simulink model "Model02"  (R2018a)
settings: Solver=VariableStepAuto  StartTime=0.0  StopTime=10.0  RelTol=1e-3
undefined symbols (not defined in the file or in its folder): b, k, m
settings Model: Creator=ameli  LastModifiedBy=ameli
settings DataIOCC: Refine=10

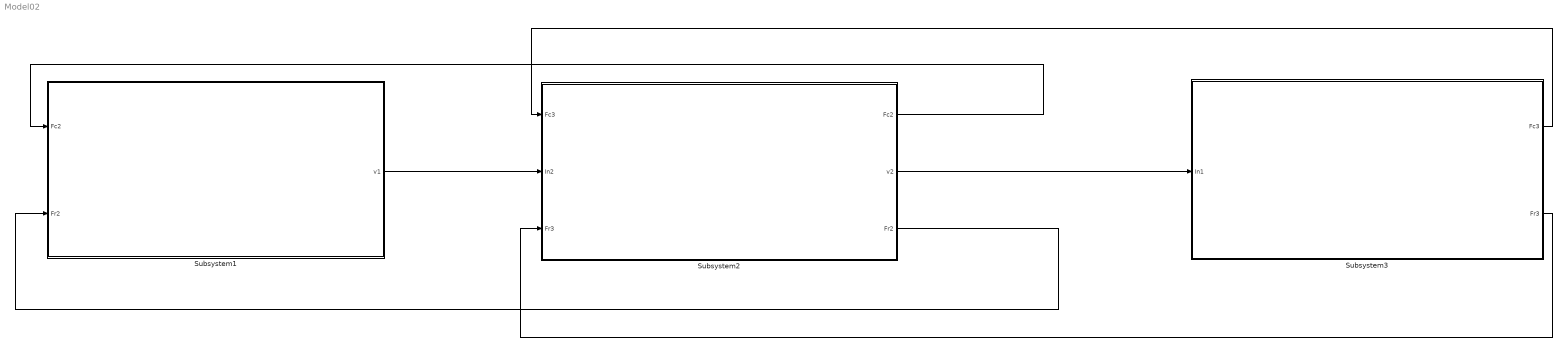
== system Model02 ==
  "Subsystem1 " : Subsystem
  Subsystem2 : Subsystem
  Subsystem3 : Subsystem
  wires:
  Subsystem3/2(Fr3) -> Subsystem2/3(Fr3)
  Subsystem2/3(Fr2) -> "Subsystem1 "/2(Fr2)
  Subsystem3/1(Fc3) -> Subsystem2/1(Fc3)
  Subsystem2/1(Fc2) -> "Subsystem1 "/1(Fc2)
  "Subsystem1 "/1(v1) -> Subsystem2/2(In2)
  Subsystem2/2(v2) -> Subsystem3/1(In1)

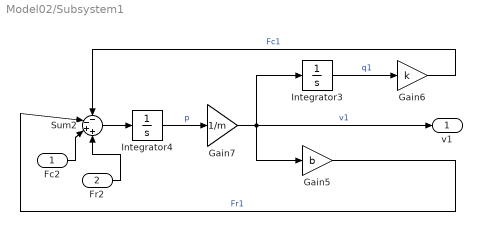
== system Model02/Subsystem1  ==
  Fc2 : Inport
  Fr2 : Inport  Port=2
  Gain5 : Gain  Gain=b
  Gain6 : Gain  Gain=k
  Gain7 : Gain  Gain=1/m
  Integrator3 : Integrator  InitialCondition=0.1
  Integrator4 : Integrator
  Sum2 : Sum  Inputs=--++
  v1 : Outport
  wires:
  Gain7/1 -> v1/1, Gain5/1, Integrator3/1  "v1"
  Gain5/1 -> Sum2/2  "Fr1"
  Integrator3/1 -> Gain6/1  "q1"
  Fr2/1 -> Sum2/4
  Integrator4/1 -> Gain7/1  "p"
  Sum2/1 -> Integrator4/1
  Gain6/1 -> Sum2/1  "Fc1"
  Fc2/1 -> Sum2/3

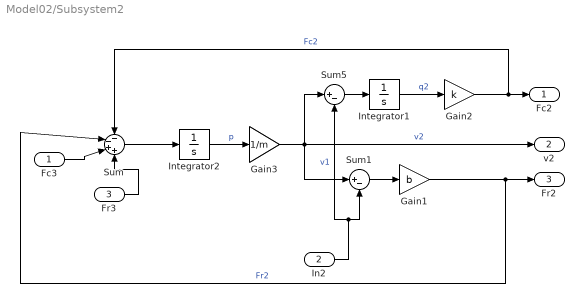
== system Model02/Subsystem2 ==
  Fc3 : Inport
  In2 : Inport  Port=2
  Fr3 : Inport  Port=3
  Gain1 : Gain  Gain=b
  Gain2 : Gain  Gain=k
  Gain3 : Gain  Gain=1/m
  Integrator1 : Integrator  InitialCondition=0.2
  Integrator2 : Integrator
  Sum : Sum  Inputs=--++
  Sum1 : Sum  Inputs=|+-
  Sum5 : Sum  Inputs=|+-
  Fc2 : Outport
  v2 : Outport  Port=2
  Fr2 : Outport  Port=3
  wires:
  Integrator2/1 -> Gain3/1  "p"
  Sum5/1 -> Integrator1/1
  Gain3/1 -> v2/1, Sum5/1, Sum1/1  "v2"
  In2/1 -> Sum5/2, Sum1/2  "v1"
  Sum/1 -> Integrator2/1
  Gain1/1 -> Sum/2, Fr2/1  "Fr2"
  Integrator1/1 -> Gain2/1  "q2"
  Gain2/1 -> Sum/1, Fc2/1  "Fc2"
  Fc3/1 -> Sum/3
  Sum1/1 -> Gain1/1
  Fr3/1 -> Sum/4

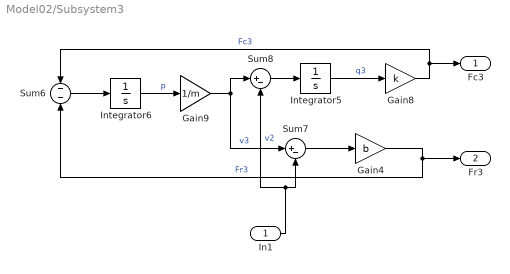
== system Model02/Subsystem3 ==
  In1 : Inport
  Gain4 : Gain  Gain=b
  Gain8 : Gain  Gain=k
  Gain9 : Gain  Gain=1/m
  Integrator5 : Integrator  InitialCondition=0.3
  Integrator6 : Integrator
  Sum6 : Sum  Inputs=--
  Sum7 : Sum  Inputs=|+-
  Sum8 : Sum  Inputs=|+-
  Fc3 : Outport
  Fr3 : Outport  Port=2
  wires:
  Sum7/1 -> Gain4/1
  Integrator6/1 -> Gain9/1  "p"
  In1/1 -> Sum8/2, Sum7/2  "v2"
  Sum6/1 -> Integrator6/1
  Gain4/1 -> Sum6/2, Fr3/1  "Fr3"
  Gain8/1 -> Fc3/1, Sum6/1  "Fc3"
  Gain9/1 -> Sum7/1, Sum8/1  "v3"
  Sum8/1 -> Integrator5/1
  Integrator5/1 -> Gain8/1  "q3"
